simulink model "Simulate_cascsaded_motor_controllers"  (R2014b)
settings: Solver=ode45  SolverMode=SingleTasking  StartTime=0.0  StopTime=10  RelTol=1e-3
values from neighbouring files (symbols this model uses):
  F_c = 1.5e-3    (= 0.0015)    [continuous_design.m]    (also in workshop1.m)
  J1 = 0.0006    [continuous_design.m]    (also in workshop1.m)
  motor = motor_pars    [continuous_design.m]    (also in workshop1.m)
  n = 5    [continuous_design.m]    (also in workshop1.m)
  R_sim = Rd.num{1}    [pbutest.m]    (also in workshop1.m)
  S_sim = Sd.num{1}    [pbutest.m]    (also in workshop1.m)
  T_sim = Td.num{1}    [pbutest.m]    (also in workshop1.m)
  Ts = 2*pi/ws    [continuous_design.m]    (also in pbutest.m = 0.0108705628152; workshop1.m = 0.108705628152)
libraries: simulink x1
settings Model: Creator=Gabriel  LastModifiedBy=es2lab2
settings OptimizationCC: BlockReduction=off  BooleanDataType=off  UseDivisionForNetSlopeComputation=off  SimCompilerOptimization=off
settings DebuggingCC: SaveWithParameterizedLinksMsg=none  UnderspecifiedInitializationDetection=Classic  MergeDetectMultiDrivingBlocksExec=none  SignalResolutionControl=TryResolveAllWithWarning  SolverPrmCheckMsg=none  FrameProcessingCompatibilityMsg=error  AllowSymbolicDim=off
settings HardwareCC: TargetUnknown=on
settings RTWCC: RTWCompilerOptimization=off
settings ConfigComp: CovMetricSettings=dw  CovHtmlReporting=on  CovSaveCumulativeToWorkspaceVar=on  CovSaveSingleToWorkspaceVar=on  CovModelRefEnable=Off  CovExternalEMLEnable=off  CovSFcnEnable=off

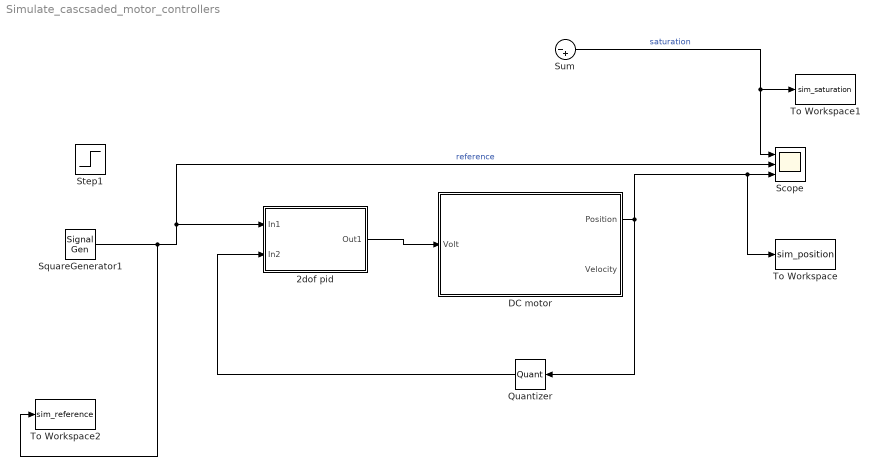
== system Simulate_cascsaded_motor_controllers ==
  2dof pid : Subsystem
  DC motor : Subsystem
  Quantizer : Quantizer  QuantizationInterval=quant
  Scope : Scope  NumInputPorts=3
      settings: TimeRange=7.551351351351352  YMin=-25.9388~-0.63233~-5  YMax=11.2811~5.69093~5
  SquareGenerator1 : SignalGenerator  WaveForm=square  Amplitude=4  Units=rad/sec
  Step1 : Step  Time=0  After=4  SampleTime=0
  Sum : Sum  Inputs=|-+
  To Workspace : ToWorkspace  VariableName=sim_position  SaveFormat=Timeseries  SampleTime=-1
  To Workspace1 : ToWorkspace  VariableName=sim_saturation  SaveFormat=Timeseries  SampleTime=-1
  To Workspace2 : ToWorkspace  VariableName=sim_reference  SaveFormat=Timeseries  SampleTime=-1
  wires:
  SquareGenerator1/1 -> To Workspace2/1, 2dof pid/1(In1), Scope/2  "reference"
  Sum/1 -> To Workspace1/1, Scope/1  "saturation"
  DC motor/1(Position) -> Quantizer/1, To Workspace/1, Scope/3
  Quantizer/1 -> 2dof pid/2(In2)
  2dof pid/1(Out1) -> DC motor/1(Volt)

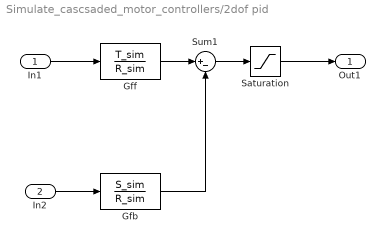
== system Simulate_cascsaded_motor_controllers/2dof pid ==
  In1 : Inport
  In2 : Inport  Port=2
  Gfb : DiscreteTransferFcn  Numerator=S_sim  Denominator=R_sim  SampleTime=Ts
  Gff : DiscreteTransferFcn  Numerator=T_sim  Denominator=R_sim  SampleTime=Ts
  Saturation : Saturate  UpperLimit=24  LowerLimit=-24
  Sum1 : Sum  Inputs=|+-
  Out1 : Outport
  wires:
  Sum1/1 -> Saturation/1
  Gfb/1 -> Sum1/2
  Saturation/1 -> Out1/1
  Gff/1 -> Sum1/1
  In1/1 -> Gff/1
  In2/1 -> Gfb/1

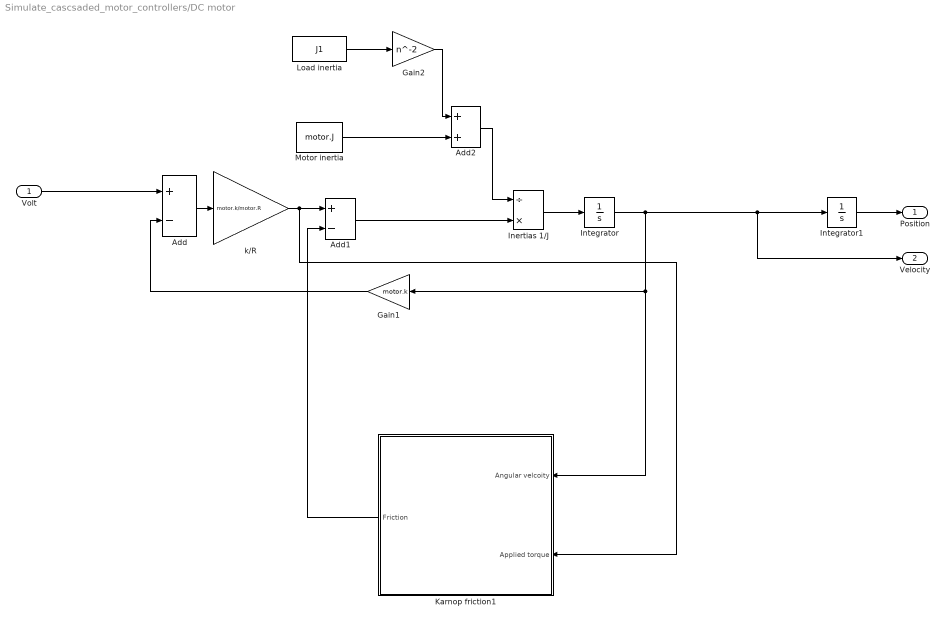
== system Simulate_cascsaded_motor_controllers/DC motor ==
  Volt : Inport
  Add : Sum  Inputs=+-
  Add1 : Sum  Inputs=+-
  Add2 : Sum
  Gain1 : Gain  Gain=motor.k
  Gain2 : Gain  Gain=n^-2
  Inertias 1/J : Product  Inputs=/*
  Integrator : Integrator
  Integrator1 : Integrator
  Karnop friction1 : Subsystem
  Load inertia : Constant  Value=J1
  Motor inertia : Constant  Value=motor.J
  "k/R " : Gain  Gain=motor.k/motor.R
  Position : Outport
  Velocity : Outport  Port=2
  wires:
  Karnop friction1/1(Friction) -> Add1/2
  Add2/1 -> Inertias 1/J/1
  Gain2/1 -> Add2/1
  Load inertia/1 -> Gain2/1
  Motor inertia/1 -> Add2/2
  Integrator/1 -> Integrator1/1, Velocity/1, Karnop friction1/1(Angular velcoity), Gain1/1
  Volt/1 -> Add/1
  Add1/1 -> Inertias 1/J/2
  Integrator1/1 -> Position/1
  Inertias 1/J/1 -> Integrator/1
  "k/R "/1 -> Add1/1, Karnop friction1/2(Applied torque)
  Add/1 -> "k/R "/1
  Gain1/1 -> Add/2

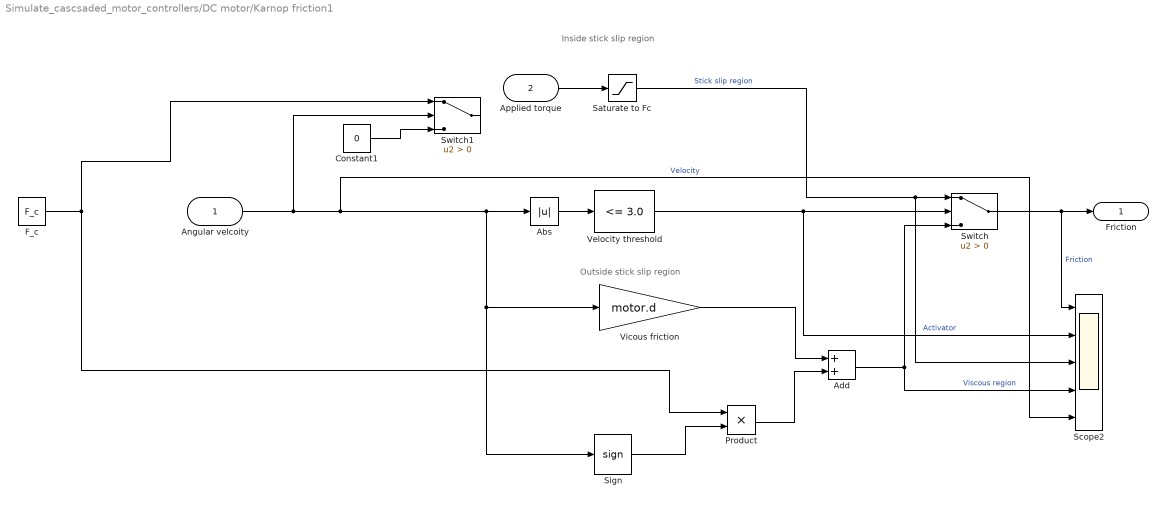
== system Simulate_cascsaded_motor_controllers/DC motor/Karnop friction1 ==
  note: Outside stick slip region
  note: Inside stick slip region
  Angular velcoity : Inport
  Applied torque : Inport  Port=2
  Abs : Abs  ZeroCross=off
  Add : Sum
  Constant1 : Constant  Value=0
  F_c : Constant  Value=F_c
  Product : Product
  Saturate to Fc : Saturate  UpperLimit=F_c  LowerLimit=-F_c  ZeroCross=off
  Scope2 : Scope  NumInputPorts=5
  Sign : Signum  ZeroCross=off
  Switch : Switch  Criteria=u2 > Threshold  ZeroCross=off
  Switch1 : Switch  Criteria=u2 > Threshold  ZeroCross=off
  "Velocity threshold " : simulink/Logic and Bit Operations/Compare To Constant  relop=<=  const=3.0  OutDataTypeStr=boolean
  Vicous friction : Gain  Gain=motor.d
  Friction : Outport
  wires:
  Applied torque/1 -> Saturate to Fc/1
  Add/1 -> Scope2/4, Switch/3  "Viscous region"
  Sign/1 -> Product/2
  F_c/1 -> Product/1, Switch1/1
  Vicous friction/1 -> Add/1
  Product/1 -> Add/2
  Abs/1 -> "Velocity threshold "/1
  "Velocity threshold "/1 -> Switch/2, Scope2/2  "Activator"
  Angular velcoity/1 -> Switch1/2, Sign/1, Vicous friction/1, Abs/1, Scope2/5  "Velocity"
  Switch/1 -> Friction/1, Scope2/1  "Friction"
  Saturate to Fc/1 -> Switch/1, Scope2/3  "Stick slip region"
  Constant1/1 -> Switch1/3
